simulink model "nuri3s_computed_torque_PD"  (R2024b)
settings: Solver=VariableStepAuto  StartTime=0.0  StopTime=5  RelTol=1e-3
undefined symbols (not defined in the file): q_goal_rad, q_start, robot
libraries: robotmaniplib x2, robotcorelib x1
settings Model: Creator=user  LastModifiedBy=변재형

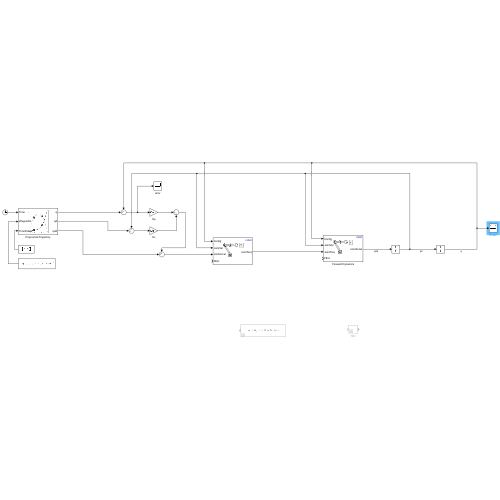
[thumbnail: Simulink's stored preview of the top-level diagram]
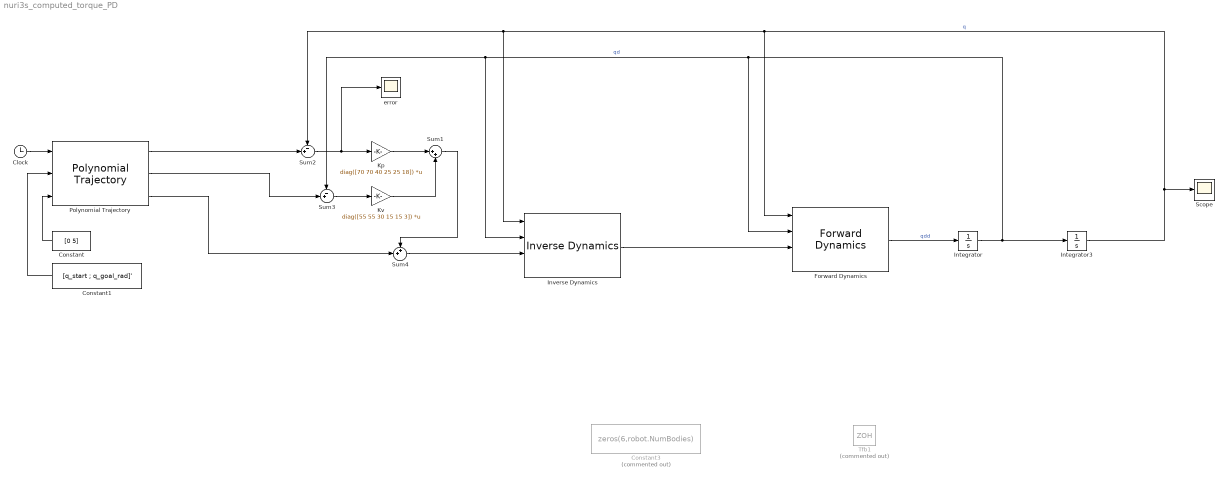
== system nuri3s_computed_torque_PD ==
  Clock : Clock
  Constant : Constant  Value=[0 5]
  Constant1 : Constant  Value=[q_start ; q_goal_rad]'
  Constant3 : Constant  Commented=on  Value=zeros(6,robot.NumBodies)
  Forward Dynamics : robotmaniplib/Forward Dynamics  RigidBodyTree=robot  SimulateUsing=Interpreted execution
  Integrator : Integrator
  Integrator3 : Integrator
  Inverse Dynamics : robotmaniplib/Inverse Dynamics  RigidBodyTree=robot  SimulateUsing=Interpreted execution
  Kp : Gain  Gain=diag([70 70 40 25 25 18])  Multiplication=Matrix(K*u)
  Kv : Gain  Gain=diag([55 55 30 15 15 3])  Multiplication=Matrix(K*u)
  Polynomial Trajectory : robotcorelib/Polynomial Trajectory  WaypointSource=External  Waypoints=[ 0, 2, 1, 5, 0; -1, 3, 1, 4, 4 ]  TimePoints=[ 0, 1, 2, 3, 4 ]  TimeInterval=[ 1, 4 ]  Method=Quintic Polynomial  ParameterSource=Internal  VelocityBoundaryCondition=zeros( 6, 2 )  AccelerationBoundaryCondition=zeros( 6, 2 )  SimulateUsing=Interpreted execution
  Scope : Scope
  Sum1 : Sum  Inputs=|++
  Sum2 : Sum  Inputs=-+|
  Sum3 : Sum  Inputs=-+|
  Sum4 : Sum  Inputs=++|
  Tfb1 : ZeroOrderHold  Commented=on  SampleTime=0.001
  error : Scope
  wires:
  Forward Dynamics/1 -> Integrator/1  "qdd"
  Integrator/1 -> Integrator3/1, Forward Dynamics/2, Inverse Dynamics/2, Sum3/1  "qd"
  Integrator3/1 -> Scope/1, Forward Dynamics/1, Inverse Dynamics/1, Sum2/1  "q"
  Clock/1 -> Polynomial Trajectory/1
  Constant/1 -> Polynomial Trajectory/3
  Constant1/1 -> Polynomial Trajectory/2
  Kp/1 -> Sum1/1
  Sum3/1 -> Kv/1
  Sum2/1 -> Kp/1, error/1
  Sum4/1 -> Inverse Dynamics/3
  Polynomial Trajectory/1 -> Sum2/2
  Polynomial Trajectory/2 -> Sum3/2
  Polynomial Trajectory/3 -> Sum4/2
  Sum1/1 -> Sum4/1
  Kv/1 -> Sum1/2
  Inverse Dynamics/1 -> Forward Dynamics/3
